simulink model "ScriptDemo"  (R2022b)
settings: configuration reference "TmVcThermal_Configuration_sub" (kept outside this file)
undefined symbols (not defined in the file or in its folder): aaaa, bbbb, cTmComprCtrl_D_u8HvacFlowTable_db, cTmComprCtrl_D_u8HvacFlowTable_sw, cTmComprCtrl_n_i16ChillCmpIMax, cTmComprCtrl_n_i16ChillCmpIMin, cTmComprCtrl_n_i16ChillCmpIMin666, cTmComprCtrl_n_i16ChillCmpPMax, cTmComprCtrl_n_i16ChillCmpPMin, cTmComprCtrl_n_i16CmpChillCoolRpmKiMax, cTmComprCtrl_n_i16CmpChillCoolRpmKiMin, cTmComprCtrl_n_i16CmpChillCoolRpmKpMax, cTmComprCtrl_n_i16CmpChillCoolRpmKpMin, cTmComprCtrl_n_i16CmpCoolRpmKiMax, cTmComprCtrl_n_i16CmpCoolRpmKiMin, cTmComprCtrl_n_i16CmpCoolRpmKpMax, cTmComprCtrl_n_i16CmpCoolRpmKpMin, cTmComprCtrl_n_i16SM4CmpHeatKiMax, cTmComprCtrl_n_i16SM4CmpHeatKiMin, cTmComprCtrl_n_i16SM4CmpHeatKpMax, cTmComprCtrl_n_i16SM4CmpHeatKpMin, cTmComprCtrl_n_i16SM5CmpHeatKiMax, cTmComprCtrl_n_i16SM5CmpHeatKiMin, cTmComprCtrl_n_i16SM5CmpHeatKpMax, cTmComprCtrl_n_i16SM5CmpHeatKpMin, cTmComprCtrl_n_i16SM6CmpHeatKiMax, cTmComprCtrl_n_i16SM6CmpHeatKiMin, cTmComprCtrl_n_i16SM6CmpHeatKpMax, cTmComprCtrl_n_i16SM6CmpHeatKpMin, cTmComprCtrl_n_u16CmpMaxSpdFanFltLimt, cTmComprCtrl_n_u16CmpMaxSpdLoSidePFltLimt, cTmComprCtrl_n_u16CmpMaxSpdSensorFltLimt, cTmComprCtrl_n_u16CompMinRpm, cTmComprCtrl_n_u16CompRpmIncThres, cTmComprCtrl_t_u16BattCooltFFPeriod, cTmComprCtrl_t_u16BattCooltPIPeriod, cTmComprCtrl_t_u16CmpCoolFFPeriod, cTmComprCtrl_t_u16CmpCoolPIPeriod, cTmComprCtrl_t_u16CoolCmpChillFFPeriod, cTmComprCtrl_t_u16CoolCmpChillPIPeriod, cTmComprCtrl_t_u16SM4CmpHeatFFPeriod, cTmComprCtrl_t_u16SM4CmpHeatPIPeriod, cTmComprCtrl_t_u16SM5CmpHeatFFPeriod, cTmComprCtrl_t_u16SM5CmpHeatPIPeriod, cTmComprCtrl_t_u16SM6CmpHeatFFPeriod, cTmComprCtrl_t_u16SM6CmpHeatPIPeriod, cTmComprCtrl_Te_EvapClearInteg, cTmComprCtrl_Te_i16HpReqTempSaturoffset, cTmComprCtrl_Te_i16SatLpReplaceDiff, cTmComprCtrl_Te_i16SM3BatDiffStartEvapDecOffset, cTmComprCtrl_Te_i16SM3EvapLo, cTmComprCtrl_Te_i16SM3TBatDiffEntEvapDecOffset, cTmComprCtrl_Te_i16SM3TBatDiffEntEvapDecOffsetQuit, cTmComprCtrl_Te_s32ErrCmpChillPIContinueCoolH, cTmComprCtrl_Te_s32ErrCmpChillPIContinueCoolL, cTmComprCtrl_Te_s32ErrCmpPIContinueChillH, cTmComprCtrl_Te_s32ErrCmpPIContinueChillL, cTmComprCtrl_Te_s32ErrCmpPIContinueCoolH, cTmComprCtrl_Te_s32ErrCmpPIContinueCoolL, cTmComprCtrl_Te_s32ErrCmpPIContinueHeatH ... (+398)
libraries: simulink x846, PCMULib x711, simulink_need_slupdate x4
(part 4 of 49)

== system ScriptDemo/Create/creatIFIn/After ==
  note: % 目的: 创建接口输入模型
      | % 限制: 本函数仅仅用于热系统autosar 系统， 运行函数前，需要提前加载生成arxml 对应的IDT文件
      | % 范例：creatIFIn('sheetNames',{'IF_InportsCommon','IF_InportsDiag','IF_Inports2F'})
  sVcCcm_Te_AmbTEstimd : Inport  OutputFunctionCall=on
  yVcCcm_B_AmbTEstimdQf : Inport  Port=2  OutDataTypeStr=boolean
  sVcCcm_Te_IncarTemp : Inport  Port=3
  sVcCcm_Qf_IncarTempQf : Inport  Port=4
  sVcCcm_Te_Evap : Inport  Port=5
  sVcCcm_Qf_TeEvap : Inport  Port=6
  yVcCcm_B_AirCondEnbl : Inport  Port=7  OutDataTypeStr=boolean
  sVcCcm_Te_EvapReq : Inport  Port=8
  yVcCcm_B_HvacHeatgReq : Inport  Port=9  OutDataTypeStr=boolean
  sVcCcm_Z_HvacAirMFlowEstimd : Inport  Port=10
  sVcCcm_Z_HexHeatrAirMFlowEstimd : Inport  Port=11
  sVcCcm_D_HvacFanSts : Inport  Port=12
  sVcCcm_X_ClimtRcirc : Inport  Port=13
  sVcCcm_X_HvacTFlpActlPosnFrtRowLe : Inport  Port=14
  sVcCcm_X_HvacTFlpActlPosnFrtRowRi : Inport  Port=15
  sVcCcm_Te_HeatrAirTReq : Inport  Port=16
  sVcCcm_Te_HvacHexAirT : Inport  Port=17
  yVcCcm_B_HvacHexAirTQf : Inport  Port=18  OutDataTypeStr=boolean
  yVcVdm_B_EcoClimaSts : Inport  Port=19  OutDataTypeStr=boolean
  Event_DTC_126A12_GetEventStatus : Inport  Port=20
  Event_DTC_126A14_GetEventStatus : Inport  Port=21
  Event_DTC_124314_GetEventStatus : Inport  Port=22
  Event_DTC_124312_GetEventStatus : Inport  Port=23
  Event_DTC_128D11_GetEventStatus : Inport  Port=24
  Event_DTC_128D15_GetEventStatus : Inport  Port=25
  Event_DTC_507011_GetEventStatus : Inport  Port=26
  Event_DTC_507015_GetEventStatus : Inport  Port=27
  Event_DTC_507111_GetEventStatus : Inport  Port=28
  Event_DTC_507115_GetEventStatus : Inport  Port=29
  Event_DTC_507C11_GetEventStatus : Inport  Port=30
  Event_DTC_507C15_GetEventStatus : Inport  Port=31
  Event_DTC_508C11_GetEventStatus : Inport  Port=32
  Event_DTC_508C15_GetEventStatus : Inport  Port=33
  Event_DTC_0A0011_GetEventStatus : Inport  Port=34
  Event_DTC_0A0015_GetEventStatus : Inport  Port=35
  Event_DTC_131F9C_GetEventStatus : Inport  Port=36
  Event_DTC_10687A_GetEventStatus : Inport  Port=37
  Event_DTC_91FF12_GetEventStatus : Inport  Port=38
  Event_DTC_91FF14_GetEventStatus : Inport  Port=39
  yGlAcHpM_B_HpmSov1Actv2FReq : Inport  Port=40  OutDataTypeStr=boolean
  yGlAcHpM_B_HpmSov1ActvCmd2F : Inport  Port=41  OutDataTypeStr=boolean
  yGlAcHpM_B_HpmSov2Actv2FReq : Inport  Port=42  OutDataTypeStr=boolean
  yGlAcHpM_B_HpmSov2ActvCmd2F : Inport  Port=43  OutDataTypeStr=boolean
  yGlAcHpM_B_HpmSov3Actv2FReq : Inport  Port=44  OutDataTypeStr=boolean
  yGlAcHpM_B_HpmSov3ActvCmd2F : Inport  Port=45  OutDataTypeStr=boolean
  yVcEac_B_ChillerValve2FReq : Inport  Port=46  OutDataTypeStr=boolean
  yVcEac_B_ChillerValveReq2F : Inport  Port=47  OutDataTypeStr=boolean
  yVcAc_B_EvaprVlvFrnt2FReq : Inport  Port=48  OutDataTypeStr=boolean
  yVcAc_B_EvaprVlvReqFrnt2F : Inport  Port=49  OutDataTypeStr=boolean
  yVcTmAf_B_FanPwm2FReq : Inport  Port=50  OutDataTypeStr=boolean
  sVcTmAf_X_FanPwmReq2F : Inport  Port=51
  yGlTmHgMgt_B_PTCPumpSpd2FReq : Inport  Port=52  OutDataTypeStr=boolean
  sGlTmHgMgt_X_PTCPumpSpdReq2F : Inport  Port=53
  yGlHwDrvDiag_B_BattPmp2FReq : Inport  Port=54  OutDataTypeStr=boolean
  sGlTmBcc_X_BattCooltPmpReq2F : Inport  Port=55
  yVcTmHcc_B_EmCooltPmp2FReq : Inport  Port=56  OutDataTypeStr=boolean
  sVcTmHcc_X_EmCooltPmpReq2F : Inport  Port=57
  yVcBctv_B_VlvPos2FReq : Inport  Port=58  OutDataTypeStr=boolean
  sVcBctv_X_VlvPosReq2F : Inport  Port=59
  TmIn : Subsystem
  wires:
  TmIn/1(sTmIn_Te_s32AmbTEstimd) -> [sTmIn_Te_s32AmbTEstimd]
  TmIn/2(yTmIn_B_AmbTEstimdQf) -> [yTmIn_B_AmbTEstimdQf]
  TmIn/3(sTmIn_Te_s32IncarTemp) -> [sTmIn_Te_s32IncarTemp]
  TmIn/4(sTmIn_D_u8IncarTempQf) -> [sTmIn_D_u8IncarTempQf]
  TmIn/5(sTmIn_Te_s32Evap) -> [sTmIn_Te_s32Evap]
  TmIn/6(yTmIn_B_TeEvap) -> [yTmIn_B_TeEvap]
  TmIn/7(yTmIn_B_AirCondEnbl) -> [yTmIn_B_AirCondEnbl]
  TmIn/8(sTmIn_Te_s32EvapReq) -> [sTmIn_Te_s32EvapReq]
  TmIn/9(yTmIn_B_HvacHeatgReq) -> [yTmIn_B_HvacHeatgReq]
  TmIn/10(sTmIn_md_s32HvacAirMFlowEstimd) -> [sTmIn_md_s32HvacAirMFlowEstimd]
  TmIn/11(sTmIn_md_s32HexHeatrAirMFlowEstimd) -> [sTmIn_md_s32HexHeatrAirMFlowEstimd]
  TmIn/12(sTmIn_D_u8HvacFanSts) -> [sTmIn_D_u8HvacFanSts]
  TmIn/13(sTmIn_X_s32ClimtRcirc) -> [sTmIn_X_s32ClimtRcirc]
  TmIn/14(sTmIn_X_s32HvacTFlpActlPosnFrtRowLe) -> [sTmIn_X_s32HvacTFlpActlPosnFrtRowLe]
  TmIn/15(sTmIn_X_s32HvacTFlpActlPosnFrtRowRi) -> [sTmIn_X_s32HvacTFlpActlPosnFrtRowRi]
  TmIn/16(sTmIn_Te_s32HeatrAirTReq) -> [sTmIn_Te_s32HeatrAirTReq]
  TmIn/17(sTmIn_Te_s32HvacHexAirT) -> [sTmIn_Te_s32HvacHexAirT]
  TmIn/18(yTmIn_B_HvacHexAirTQf) -> [yTmIn_B_HvacHexAirTQf]
  TmIn/19(yTmIn_B_EcoClimaSts) -> [yTmIn_B_EcoClimaSts]
  TmIn/20(sTmIn_D_u8VcEvLoSidePSB) -> [sTmIn_D_u8VcEvLoSidePSB]
  TmIn/21(sTmIn_D_u8VcEvLoSidePOP) -> [sTmIn_D_u8VcEvLoSidePOP]
  TmIn/22(sTmIn_D_u8VcEvHiSidePOP) -> [sTmIn_D_u8VcEvHiSidePOP]
  TmIn/23(sTmIn_D_u8VcEvHiSidePSB) -> [sTmIn_D_u8VcEvHiSidePSB]
  TmIn/24(sTmIn_D_u8VcEvHiSideTmpSnrSG) -> [sTmIn_D_u8VcEvHiSideTmpSnrSG]
  TmIn/25(sTmIn_D_u8VcEvOutrCondOutTOP) -> [sTmIn_D_u8VcEvOutrCondOutTOP]
  TmIn/26(sTmIn_D_u8VcEvChillerOutTSG) -> [sTmIn_D_u8VcEvChillerOutTSG]
  TmIn/27(sTmIn_D_u8VcEvChillerOutTOP) -> [sTmIn_D_u8VcEvChillerOutTOP]
  TmIn/28(sTmIn_D_u8VcEvInrCondOutTSG) -> [sTmIn_D_u8VcEvInrCondOutTSG]
  TmIn/29(sTmIn_D_u8VcEvInrCondOutTOP) -> [sTmIn_D_u8VcEvInrCondOutTOP]
  TmIn/30(sTmIn_D_u8VcEvEvapOutTSG) -> [sTmIn_D_u8VcEvEvapOutTSG]
  TmIn/31(sTmIn_D_u8VcEvEvapOutTOP) -> [sTmIn_D_u8VcEvEvapOutTOP]
  TmIn/32(sTmIn_D_u8VcEvCmprDischrgTSG) -> [sTmIn_D_u8VcEvCmprDischrgTSG]
  TmIn/33(sTmIn_D_u8VcEvCmprDischrgTOP) -> [sTmIn_D_u8VcEvCmprDischrgTOP]
  TmIn/34(sTmIn_D_u8VcEvTmpClSrSG) -> [sTmIn_D_u8VcEvTmpClSrSG]
  TmIn/35(sTmIn_D_u8VcEvTmpClSrOP) -> [sTmIn_D_u8VcEvTmpClSrOP]
  TmIn/36(sTmIn_D_u8VcEvELDTCooltLvlLo) -> [sTmIn_D_u8VcEvELDTCooltLvlLo]
  TmIn/37(sTmIn_D_u8VcEvBattCooltLvlLo) -> [sTmIn_D_u8VcEvBattCooltLvlLo]
  TmIn/38(sTmIn_D_u8VcEvNoHpHighSidePSnrSB) -> [sTmIn_D_u8VcEvNoHpHighSidePSnrSB]
  TmIn/39(sTmIn_D_u8VcEvNoHpHighSidePSnrOP) -> [sTmIn_D_u8VcEvNoHpHighSidePSnrOP]
  TmIn/40(yTmIn_B_HpmSov1Actv2FReq) -> [yTmIn_B_HpmSov1Actv2FReq]
  TmIn/41(yTmIn_B_HpmSov1ActvCmd2F) -> [yTmIn_B_HpmSov1ActvCmd2F]
  TmIn/42(yTmIn_B_HpmSov2Actv2FReq) -> [yTmIn_B_HpmSov2Actv2FReq]
  TmIn/43(yTmIn_B_HpmSov2ActvCmd2F) -> [yTmIn_B_HpmSov2ActvCmd2F]
  TmIn/44(yTmIn_B_HpmSov3Actv2FReq) -> [yTmIn_B_HpmSov3Actv2FReq]
  TmIn/45(yTmIn_B_HpmSov3ActvCmd2F) -> [yTmIn_B_HpmSov3ActvCmd2F]
  TmIn/46(yTmIn_B_ChillerValve2FReq) -> [yTmIn_B_ChillerValve2FReq]
  TmIn/47(yTmIn_B_ChillerValveReq2F) -> [yTmIn_B_ChillerValveReq2F]
  TmIn/48(yTmIn_B_EvaprVlvFrnt2FReq) -> [yTmIn_B_EvaprVlvFrnt2FReq]
  TmIn/49(yTmIn_B_EvaprVlvReqFrnt2F) -> [yTmIn_B_EvaprVlvReqFrnt2F]
  TmIn/50(yTmIn_B_FanPwm2FReq) -> [yTmIn_B_FanPwm2FReq]
  TmIn/51(sTmIn_X_s32FanPwmReq2F) -> [sTmIn_X_s32FanPwmReq2F]
  TmIn/52(yTmIn_B_PTCPumpSpd2FReq) -> [yTmIn_B_PTCPumpSpd2FReq]
  TmIn/53(sTmIn_X_s32PTCPumpSpdReq2F) -> [sTmIn_X_s32PTCPumpSpdReq2F]
  TmIn/54(yTmIn_B_BattPmp2FReq) -> [yTmIn_B_BattPmp2FReq]
  TmIn/55(sTmIn_X_s32BattCooltPmpReq2F) -> [sTmIn_X_s32BattCooltPmpReq2F]
  TmIn/56(yTmIn_B_EmCooltPmp2FReq) -> [yTmIn_B_EmCooltPmp2FReq]
  TmIn/57(sTmIn_X_s32EmCooltPmpReq2F) -> [sTmIn_X_s32EmCooltPmpReq2F]
  TmIn/58(yTmIn_B_BctvVlvPos2FReq) -> [yTmIn_B_BctvVlvPos2FReq]
  TmIn/59(sTmIn_X_u8BctvVlvPosReq2F) -> [sTmIn_X_u8BctvVlvPosReq2F]
  sVcCcm_Te_AmbTEstimd/1 -> TmIn/1(sVcCcm_Te_AmbTEstimd)
  yVcCcm_B_AmbTEstimdQf/1 -> TmIn/2(yVcCcm_B_AmbTEstimdQf)
  sVcCcm_Te_IncarTemp/1 -> TmIn/3(sVcCcm_Te_IncarTemp)
  sVcCcm_Qf_IncarTempQf/1 -> TmIn/4(sVcCcm_Qf_IncarTempQf)
  sVcCcm_Te_Evap/1 -> TmIn/5(sVcCcm_Te_Evap)
  sVcCcm_Qf_TeEvap/1 -> TmIn/6(sVcCcm_Qf_TeEvap)
  yVcCcm_B_AirCondEnbl/1 -> TmIn/7(yVcCcm_B_AirCondEnbl)
  sVcCcm_Te_EvapReq/1 -> TmIn/8(sVcCcm_Te_EvapReq)
  yVcCcm_B_HvacHeatgReq/1 -> TmIn/9(yVcCcm_B_HvacHeatgReq)
  sVcCcm_Z_HvacAirMFlowEstimd/1 -> TmIn/10(sVcCcm_Z_HvacAirMFlowEstimd)
  sVcCcm_Z_HexHeatrAirMFlowEstimd/1 -> TmIn/11(sVcCcm_Z_HexHeatrAirMFlowEstimd)
  sVcCcm_D_HvacFanSts/1 -> TmIn/12(sVcCcm_D_HvacFanSts)
  sVcCcm_X_ClimtRcirc/1 -> TmIn/13(sVcCcm_X_ClimtRcirc)
  sVcCcm_X_HvacTFlpActlPosnFrtRowLe/1 -> TmIn/14(sVcCcm_X_HvacTFlpActlPosnFrtRowLe)
  sVcCcm_X_HvacTFlpActlPosnFrtRowRi/1 -> TmIn/15(sVcCcm_X_HvacTFlpActlPosnFrtRowRi)
  sVcCcm_Te_HeatrAirTReq/1 -> TmIn/16(sVcCcm_Te_HeatrAirTReq)
  sVcCcm_Te_HvacHexAirT/1 -> TmIn/17(sVcCcm_Te_HvacHexAirT)
  yVcCcm_B_HvacHexAirTQf/1 -> TmIn/18(yVcCcm_B_HvacHexAirTQf)
  yVcVdm_B_EcoClimaSts/1 -> TmIn/19(yVcVdm_B_EcoClimaSts)
  Event_DTC_126A12_GetEventStatus/1 -> TmIn/20(Event_DTC_126A12_GetEventStatus)
  Event_DTC_126A14_GetEventStatus/1 -> TmIn/21(Event_DTC_126A14_GetEventStatus)
  Event_DTC_124314_GetEventStatus/1 -> TmIn/22(Event_DTC_124314_GetEventStatus)
  Event_DTC_124312_GetEventStatus/1 -> TmIn/23(Event_DTC_124312_GetEventStatus)
  Event_DTC_128D11_GetEventStatus/1 -> TmIn/24(Event_DTC_128D11_GetEventStatus)
  Event_DTC_128D15_GetEventStatus/1 -> TmIn/25(Event_DTC_128D15_GetEventStatus)
  Event_DTC_507011_GetEventStatus/1 -> TmIn/26(Event_DTC_507011_GetEventStatus)
  Event_DTC_507015_GetEventStatus/1 -> TmIn/27(Event_DTC_507015_GetEventStatus)
  Event_DTC_507111_GetEventStatus/1 -> TmIn/28(Event_DTC_507111_GetEventStatus)
  Event_DTC_507115_GetEventStatus/1 -> TmIn/29(Event_DTC_507115_GetEventStatus)
  Event_DTC_507C11_GetEventStatus/1 -> TmIn/30(Event_DTC_507C11_GetEventStatus)
  Event_DTC_507C15_GetEventStatus/1 -> TmIn/31(Event_DTC_507C15_GetEventStatus)
  Event_DTC_508C11_GetEventStatus/1 -> TmIn/32(Event_DTC_508C11_GetEventStatus)
  Event_DTC_508C15_GetEventStatus/1 -> TmIn/33(Event_DTC_508C15_GetEventStatus)
  Event_DTC_0A0011_GetEventStatus/1 -> TmIn/34(Event_DTC_0A0011_GetEventStatus)
  Event_DTC_0A0015_GetEventStatus/1 -> TmIn/35(Event_DTC_0A0015_GetEventStatus)
  Event_DTC_131F9C_GetEventStatus/1 -> TmIn/36(Event_DTC_131F9C_GetEventStatus)
  Event_DTC_10687A_GetEventStatus/1 -> TmIn/37(Event_DTC_10687A_GetEventStatus)
  Event_DTC_91FF12_GetEventStatus/1 -> TmIn/38(Event_DTC_91FF12_GetEventStatus)
  Event_DTC_91FF14_GetEventStatus/1 -> TmIn/39(Event_DTC_91FF14_GetEventStatus)
  yGlAcHpM_B_HpmSov1Actv2FReq/1 -> TmIn/40(yGlAcHpM_B_HpmSov1Actv2FReq)
  yGlAcHpM_B_HpmSov1ActvCmd2F/1 -> TmIn/41(yGlAcHpM_B_HpmSov1ActvCmd2F)
  yGlAcHpM_B_HpmSov2Actv2FReq/1 -> TmIn/42(yGlAcHpM_B_HpmSov2Actv2FReq)
  yGlAcHpM_B_HpmSov2ActvCmd2F/1 -> TmIn/43(yGlAcHpM_B_HpmSov2ActvCmd2F)
  yGlAcHpM_B_HpmSov3Actv2FReq/1 -> TmIn/44(yGlAcHpM_B_HpmSov3Actv2FReq)
  yGlAcHpM_B_HpmSov3ActvCmd2F/1 -> TmIn/45(yGlAcHpM_B_HpmSov3ActvCmd2F)
  yVcEac_B_ChillerValve2FReq/1 -> TmIn/46(yVcEac_B_ChillerValve2FReq)
  yVcEac_B_ChillerValveReq2F/1 -> TmIn/47(yVcEac_B_ChillerValveReq2F)
  yVcAc_B_EvaprVlvFrnt2FReq/1 -> TmIn/48(yVcAc_B_EvaprVlvFrnt2FReq)
  yVcAc_B_EvaprVlvReqFrnt2F/1 -> TmIn/49(yVcAc_B_EvaprVlvReqFrnt2F)
  yVcTmAf_B_FanPwm2FReq/1 -> TmIn/50(yVcTmAf_B_FanPwm2FReq)
  sVcTmAf_X_FanPwmReq2F/1 -> TmIn/51(sVcTmAf_X_FanPwmReq2F)
  yGlTmHgMgt_B_PTCPumpSpd2FReq/1 -> TmIn/52(yGlTmHgMgt_B_PTCPumpSpd2FReq)
  sGlTmHgMgt_X_PTCPumpSpdReq2F/1 -> TmIn/53(sGlTmHgMgt_X_PTCPumpSpdReq2F)
  yGlHwDrvDiag_B_BattPmp2FReq/1 -> TmIn/54(yGlHwDrvDiag_B_BattPmp2FReq)
  sGlTmBcc_X_BattCooltPmpReq2F/1 -> TmIn/55(sGlTmBcc_X_BattCooltPmpReq2F)
  yVcTmHcc_B_EmCooltPmp2FReq/1 -> TmIn/56(yVcTmHcc_B_EmCooltPmp2FReq)
  sVcTmHcc_X_EmCooltPmpReq2F/1 -> TmIn/57(sVcTmHcc_X_EmCooltPmpReq2F)
  yVcBctv_B_VlvPos2FReq/1 -> TmIn/58(yVcBctv_B_VlvPos2FReq)
  sVcBctv_X_VlvPosReq2F/1 -> TmIn/59(sVcBctv_X_VlvPosReq2F)

== system ScriptDemo/Create/creatIFIn/Before ==

== system ScriptDemo/Create/creatIFOut/After ==
  note: % 目的: 创建接口输出模型
      | % 限制: 本函数仅仅用于热系统autosar 系统， 运行函数前，需要提前加载生成arxml 对应的IDT文件
      | % 范例：creatIFOut('sheetNames',{'IF_OutportsCommon','IF_OutportsDiag','IF_Outports2F'})
  TmOut : Subsystem
  sVcEac_n_ElacCmprReq : Outport
  sVcEac_D_ElacCmprRelease : Outport  Port=2
  sVcEac_Pw_ElacCmprMax : Outport  Port=3
  sGlTmEexv_X_VlvPosReq : Outport  Port=4
  yGlTmEexv_B_PosnHeatdReq : Outport  Port=5  OutDataTypeStr=boolean
  yGlTmEexv_B_PosnCalibReq : Outport  Port=6  OutDataTypeStr=boolean
  yGlTmEexv_B_PosnMovEnable : Outport  Port=7  OutDataTypeStr=boolean
  sGlTmBexv_X_VlvPosReq : Outport  Port=8
  yGlTmBexv_B_PosnCalibReq : Outport  Port=9  OutDataTypeStr=boolean
  yGlTmBexv_B_PosnHeatdReq : Outport  Port=10  OutDataTypeStr=boolean
  yGlTmBexv_B_PosnMovEnable : Outport  Port=11  OutDataTypeStr=boolean
  sGlTmCexv_X_VlvPosReq : Outport  Port=12
  yGlTmCexv_B_PosnCalibReq : Outport  Port=13  OutDataTypeStr=boolean
  yGlTmCexv_B_PosnHeatdReq : Outport  Port=14  OutDataTypeStr=boolean
  yGlTmCexv_B_PosnMovEnable : Outport  Port=15  OutDataTypeStr=boolean
  sGlTmBctv_D_VlvRefDrvReq : Outport  Port=16
  sGlTmBctv_D_VlvActvSaveReq : Outport  Port=17
  sGlTmBctv_X_VlvPosReq : Outport  Port=18
  sGlTmBctv_D_VlvSpdLvlReq : Outport  Port=19
  sGlTmBcfv_D_VlvRefDrvReq : Outport  Port=20
  sGlTmDiag_D_EventDTC126A12 : Outport  Port=21
  sGlTmDiag_D_EventDTC126A14 : Outport  Port=22
  sGlTmDiag_D_EventDTC124314 : Outport  Port=23
  sGlTmDiag_D_EventDTC124312 : Outport  Port=24
  sGlTmDiag_D_EventDTC128D11 : Outport  Port=25
  sGlTmDiag_D_EventDTC128D15 : Outport  Port=26
  sGlTmDiag_D_EventDTC10687A : Outport  Port=27
  sGlTmDiag_D_EventDTC976612 : Outport  Port=28
  sGlTmDiag_D_EventDTC976712 : Outport  Port=29
  sGlTmDiag_D_EventDTC979012 : Outport  Port=30
  sGlTmDiag_D_EventDTC129B12 : Outport  Port=31
  sGlTmDiag_D_EventDTC979112 : Outport  Port=32
  sGlTmDiag_D_EventDTC92FE12 : Outport  Port=33
  sGlTmDiag_D_EventDTC92FE13 : Outport  Port=34
  sGlTmDiag_D_EventDTC92FE11 : Outport  Port=35
  sGlTmDiag_D_EventDTC92FEA1 : Outport  Port=36
  sGlTmDiag_D_EventDTC92FE71 : Outport  Port=37
  sGlTmDiag_D_EventDTC92FE04 : Outport  Port=38
  sGlTmDiag_D_EventDTC92A612 : Outport  Port=39
  sGlTmDiag_D_EventDTC92A613 : Outport  Port=40
  sGlAcHpM_D_HpmSov1Actv2FEnState : Outport  Port=41
  sGlAcHpM_D_HpmSov2Actv2FEnState : Outport  Port=42
  sGlAcHpM_D_HpmSov3Actv2FEnState : Outport  Port=43
  sVcTmAf_D_FanPwm2FEnState : Outport  Port=44
  sGlTmBcc_D_BattCooltPmp2FEnState : Outport  Port=45
  sVcTmHcc_D_EmCooltPmp2FEnState : Outport  Port=46
  sGlTmHgMgt_D_PTCPumpSpd2FEnState : Outport  Port=47
  sVcEctv_D_VlvMoveEna2FEnaState : Outport  Port=48
  sVcEctv_D_VlvPos2FEnaState : Outport  Port=49
  sVcBctv_D_VlvRef2FEnaState : Outport  Port=50
  sVcBctv_D_VlvPos2FEnaState : Outport  Port=51
  sVcBcfv_D_VlvRef2FEnaState : Outport  Port=52
  sVcBcfv_D_VlvPos2FEnaState : Outport  Port=53
  sVcBexv_D_ExvCal2FEnaState : Outport  Port=54
  sVcBexv_D_ExvMoveEna2FEnaState : Outport  Port=55
  sVcBexv_D_ExvPosnReq2FEnaState : Outport  Port=56
  sVcCexv_D_ExvCal2FEnaState : Outport  Port=57
  sVcCexv_D_ExvMoveEna2FEnaState : Outport  Port=58
  sVcCexv_D_ExvPosnReq2FEnaState : Outport  Port=59
  sVcEexv_D_ExvCal2FEnaState : Outport  Port=60
  wires:
  [sTmOut_n_u16ElacCmprReq] -> TmOut/1(sTmOut_n_u16ElacCmprReq)
  [sTmOut_D_u8ElacCmprRelease] -> TmOut/2(sTmOut_D_u8ElacCmprRelease)
  [sTmOut_Pw_s32ElacCmprMax] -> TmOut/3(sTmOut_Pw_s32ElacCmprMax)
  [sTmOut_X_s32EexvVlvPosReq] -> TmOut/4(sTmOut_X_s32EexvVlvPosReq)
  [yTmOut_B_EexvPosnCalibReq] -> TmOut/5(yTmOut_B_EexvPosnCalibReq)
  [yTmOut_B_EexvPosnMovEnable] -> TmOut/6(yTmOut_B_EexvPosnMovEnable)
  [sTmOut_X_s32BexvVlvPosReq] -> TmOut/7(sTmOut_X_s32BexvVlvPosReq)
  [yTmOut_B_BexvPosnCalibReq] -> TmOut/8(yTmOut_B_BexvPosnCalibReq)
  [yTmOut_B_BexvPosnMovEnable] -> TmOut/9(yTmOut_B_BexvPosnMovEnable)
  [sTmOut_X_s32CexvVlvPosReq] -> TmOut/10(sTmOut_X_s32CexvVlvPosReq)
  [yTmOut_B_CexvPosnCalibReq] -> TmOut/11(yTmOut_B_CexvPosnCalibReq)
  [yTmOut_B_CexvPosnMovEnable] -> TmOut/12(yTmOut_B_CexvPosnMovEnable)
  [sTmOut_D_u8BctvVlvRefDrvReq] -> TmOut/13(sTmOut_D_u8BctvVlvRefDrvReq)
  [sTmOut_X_u8BctvVlvPosReq] -> TmOut/14(sTmOut_X_u8BctvVlvPosReq)
  [sTmOut_D_u8BcfvVlvRefDrvReq] -> TmOut/15(sTmOut_D_u8BcfvVlvRefDrvReq)
  [sTmOut_D_u8VcEvLowSidePSnrSB] -> TmOut/16(sTmOut_D_u8VcEvLowSidePSnrSB)
  [sTmOut_D_u8VcEvLowSidePSnrOP] -> TmOut/17(sTmOut_D_u8VcEvLowSidePSnrOP)
  [sTmOut_D_u8VcEvHiSidePSnrOP] -> TmOut/18(sTmOut_D_u8VcEvHiSidePSnrOP)
  [sTmOut_D_u8VcEvHiSidePSnrSB] -> TmOut/19(sTmOut_D_u8VcEvHiSidePSnrSB)
  [sTmOut_D_u8VcEvHiSideTmpSnrSG] -> TmOut/20(sTmOut_D_u8VcEvHiSideTmpSnrSG)
  [sTmOut_D_u8VcEvHiSideTmpSnrOP] -> TmOut/21(sTmOut_D_u8VcEvHiSideTmpSnrOP)
  [sTmOut_D_u8VcEvBattCooltLvlLo] -> TmOut/22(sTmOut_D_u8VcEvBattCooltLvlLo)
  [sTmOut_D_u8VcEvSov1SB] -> TmOut/23(sTmOut_D_u8VcEvSov1SB)
  [sTmOut_D_u8VcEvSov2SB] -> TmOut/24(sTmOut_D_u8VcEvSov2SB)
  [sTmOut_D_u8VcEvSov3SB] -> TmOut/25(sTmOut_D_u8VcEvSov3SB)
  [sTmOut_D_u8VcEvSov5SB] -> TmOut/26(sTmOut_D_u8VcEvSov5SB)
  [sTmOut_D_u8VcEvSov4SB] -> TmOut/27(sTmOut_D_u8VcEvSov4SB)
  [sTmOut_D_u8VcEvSBFan] -> TmOut/28(sTmOut_D_u8VcEvSBFan)
  [sTmOut_D_u8VcEvOPFan] -> TmOut/29(sTmOut_D_u8VcEvOPFan)
  [sTmOut_D_u8VcEvSGFan] -> TmOut/30(sTmOut_D_u8VcEvSGFan)
  [sTmOut_D_u8VcEvVolErrFan] -> TmOut/31(sTmOut_D_u8VcEvVolErrFan)
  [sTmOut_D_u8VcEvBlokFan] -> TmOut/32(sTmOut_D_u8VcEvBlokFan)
  [sTmOut_D_u8VcEvCircutInteFlt] -> TmOut/33(sTmOut_D_u8VcEvCircutInteFlt)
  [sTmOut_D_u8VcEvHmPumpSB] -> TmOut/34(sTmOut_D_u8VcEvHmPumpSB)
  [sTmOut_D_u8VcEvHmPumpOC] -> TmOut/35(sTmOut_D_u8VcEvHmPumpOC)
  [sTmOut_D_u8HpmSov1Actv2FEnState] -> TmOut/36(sTmOut_D_u8HpmSov1Actv2FEnState)
  [sTmOut_D_u8HpmSov2Actv2FEnState] -> TmOut/37(sTmOut_D_u8HpmSov2Actv2FEnState)
  [sTmOut_D_u8HpmSov3Actv2FEnState] -> TmOut/38(sTmOut_D_u8HpmSov3Actv2FEnState)
  [sTmOut_D_u8FanPwm2FEnState] -> TmOut/39(sTmOut_D_u8FanPwm2FEnState)
  [sTmOut_D_u8BattCooltPmp2FEnState] -> TmOut/40(sTmOut_D_u8BattCooltPmp2FEnState)
  [sTmOut_D_u8EmCooltPmp2FEnState] -> TmOut/41(sTmOut_D_u8EmCooltPmp2FEnState)
  [sTmOut_D_u8PTCPumpSpd2FEnState] -> TmOut/42(sTmOut_D_u8PTCPumpSpd2FEnState)
  [sTmOut_D_u8EctvVlvMoveEna2FEnaState] -> TmOut/43(sTmOut_D_u8EctvVlvMoveEna2FEnaState)
  [sTmOut_D_u8EctvVlvPos2FEnaState] -> TmOut/44(sTmOut_D_u8EctvVlvPos2FEnaState)
  [sTmOut_D_u8BctvVlvRef2FEnaState] -> TmOut/45(sTmOut_D_u8BctvVlvRef2FEnaState)
  [sTmOut_D_u8BctvVlvPos2FEnaState] -> TmOut/46(sTmOut_D_u8BctvVlvPos2FEnaState)
  [sTmOut_D_u8BcfvVlvRef2FEnaState] -> TmOut/47(sTmOut_D_u8BcfvVlvRef2FEnaState)
  [sTmOut_D_u8BcfvVlvPos2FEnaState] -> TmOut/48(sTmOut_D_u8BcfvVlvPos2FEnaState)
  [sTmOut_D_u8BexvCal2FEnaState] -> TmOut/49(sTmOut_D_u8BexvCal2FEnaState)
  [sTmOut_D_u8BexvMoveEna2FEnaState] -> TmOut/50(sTmOut_D_u8BexvMoveEna2FEnaState)
  [sTmOut_D_u8BexvPosnReq2FEnaState] -> TmOut/51(sTmOut_D_u8BexvPosnReq2FEnaState)
  [sTmOut_D_u8CexvCal2FEnaState] -> TmOut/52(sTmOut_D_u8CexvCal2FEnaState)
  [sTmOut_D_u8CexvMoveEna2FEnaState] -> TmOut/53(sTmOut_D_u8CexvMoveEna2FEnaState)
  [sTmOut_D_u8CexvPosnReq2FEnaState] -> TmOut/54(sTmOut_D_u8CexvPosnReq2FEnaState)
  [sTmOut_D_u8EexvCal2FEnaState] -> TmOut/55(sTmOut_D_u8EexvCal2FEnaState)
  TmOut/1(sVcEac_n_ElacCmprReq) -> sVcEac_n_ElacCmprReq/1
  TmOut/2(sVcEac_D_ElacCmprRelease) -> sVcEac_D_ElacCmprRelease/1
  TmOut/3(sVcEac_Pw_ElacCmprMax) -> sVcEac_Pw_ElacCmprMax/1
  TmOut/4(sGlTmEexv_X_VlvPosReq) -> sGlTmEexv_X_VlvPosReq/1
  TmOut/5(yGlTmEexv_B_PosnHeatdReq) -> yGlTmEexv_B_PosnHeatdReq/1
  TmOut/6(yGlTmEexv_B_PosnCalibReq) -> yGlTmEexv_B_PosnCalibReq/1
  TmOut/7(yGlTmEexv_B_PosnMovEnable) -> yGlTmEexv_B_PosnMovEnable/1
  TmOut/8(sGlTmBexv_X_VlvPosReq) -> sGlTmBexv_X_VlvPosReq/1
  TmOut/9(yGlTmBexv_B_PosnCalibReq) -> yGlTmBexv_B_PosnCalibReq/1
  TmOut/10(yGlTmBexv_B_PosnHeatdReq) -> yGlTmBexv_B_PosnHeatdReq/1
  TmOut/11(yGlTmBexv_B_PosnMovEnable) -> yGlTmBexv_B_PosnMovEnable/1
  TmOut/12(sGlTmCexv_X_VlvPosReq) -> sGlTmCexv_X_VlvPosReq/1
  TmOut/13(yGlTmCexv_B_PosnCalibReq) -> yGlTmCexv_B_PosnCalibReq/1
  TmOut/14(yGlTmCexv_B_PosnHeatdReq) -> yGlTmCexv_B_PosnHeatdReq/1
  TmOut/15(yGlTmCexv_B_PosnMovEnable) -> yGlTmCexv_B_PosnMovEnable/1
  TmOut/16(sGlTmBctv_D_VlvRefDrvReq) -> sGlTmBctv_D_VlvRefDrvReq/1
  TmOut/17(sGlTmBctv_D_VlvActvSaveReq) -> sGlTmBctv_D_VlvActvSaveReq/1
  TmOut/18(sGlTmBctv_X_VlvPosReq) -> sGlTmBctv_X_VlvPosReq/1
  TmOut/19(sGlTmBctv_D_VlvSpdLvlReq) -> sGlTmBctv_D_VlvSpdLvlReq/1
  TmOut/20(sGlTmBcfv_D_VlvRefDrvReq) -> sGlTmBcfv_D_VlvRefDrvReq/1
  TmOut/21(sGlTmDiag_D_EventDTC126A12) -> sGlTmDiag_D_EventDTC126A12/1
  TmOut/22(sGlTmDiag_D_EventDTC126A14) -> sGlTmDiag_D_EventDTC126A14/1
  TmOut/23(sGlTmDiag_D_EventDTC124314) -> sGlTmDiag_D_EventDTC124314/1
  TmOut/24(sGlTmDiag_D_EventDTC124312) -> sGlTmDiag_D_EventDTC124312/1
  TmOut/25(sGlTmDiag_D_EventDTC128D11) -> sGlTmDiag_D_EventDTC128D11/1
  TmOut/26(sGlTmDiag_D_EventDTC128D15) -> sGlTmDiag_D_EventDTC128D15/1
  TmOut/27(sGlTmDiag_D_EventDTC10687A) -> sGlTmDiag_D_EventDTC10687A/1
  TmOut/28(sGlTmDiag_D_EventDTC976612) -> sGlTmDiag_D_EventDTC976612/1
  TmOut/29(sGlTmDiag_D_EventDTC976712) -> sGlTmDiag_D_EventDTC976712/1
  TmOut/30(sGlTmDiag_D_EventDTC979012) -> sGlTmDiag_D_EventDTC979012/1
  TmOut/31(sGlTmDiag_D_EventDTC129B12) -> sGlTmDiag_D_EventDTC129B12/1
  TmOut/32(sGlTmDiag_D_EventDTC979112) -> sGlTmDiag_D_EventDTC979112/1
  TmOut/33(sGlTmDiag_D_EventDTC92FE12) -> sGlTmDiag_D_EventDTC92FE12/1
  TmOut/34(sGlTmDiag_D_EventDTC92FE13) -> sGlTmDiag_D_EventDTC92FE13/1
  TmOut/35(sGlTmDiag_D_EventDTC92FE11) -> sGlTmDiag_D_EventDTC92FE11/1
  TmOut/36(sGlTmDiag_D_EventDTC92FEA1) -> sGlTmDiag_D_EventDTC92FEA1/1
  TmOut/37(sGlTmDiag_D_EventDTC92FE71) -> sGlTmDiag_D_EventDTC92FE71/1
  TmOut/38(sGlTmDiag_D_EventDTC92FE04) -> sGlTmDiag_D_EventDTC92FE04/1
  TmOut/39(sGlTmDiag_D_EventDTC92A612) -> sGlTmDiag_D_EventDTC92A612/1
  TmOut/40(sGlTmDiag_D_EventDTC92A613) -> sGlTmDiag_D_EventDTC92A613/1
  TmOut/41(sGlAcHpM_D_HpmSov1Actv2FEnState) -> sGlAcHpM_D_HpmSov1Actv2FEnState/1
  TmOut/42(sGlAcHpM_D_HpmSov2Actv2FEnState) -> sGlAcHpM_D_HpmSov2Actv2FEnState/1
  TmOut/43(sGlAcHpM_D_HpmSov3Actv2FEnState) -> sGlAcHpM_D_HpmSov3Actv2FEnState/1
  TmOut/44(sVcTmAf_D_FanPwm2FEnState) -> sVcTmAf_D_FanPwm2FEnState/1
  TmOut/45(sGlTmBcc_D_BattCooltPmp2FEnState) -> sGlTmBcc_D_BattCooltPmp2FEnState/1
  TmOut/46(sVcTmHcc_D_EmCooltPmp2FEnState) -> sVcTmHcc_D_EmCooltPmp2FEnState/1
  TmOut/47(sGlTmHgMgt_D_PTCPumpSpd2FEnState) -> sGlTmHgMgt_D_PTCPumpSpd2FEnState/1
  TmOut/48(sVcEctv_D_VlvMoveEna2FEnaState) -> sVcEctv_D_VlvMoveEna2FEnaState/1
  TmOut/49(sVcEctv_D_VlvPos2FEnaState) -> sVcEctv_D_VlvPos2FEnaState/1
  TmOut/50(sVcBctv_D_VlvRef2FEnaState) -> sVcBctv_D_VlvRef2FEnaState/1
  TmOut/51(sVcBctv_D_VlvPos2FEnaState) -> sVcBctv_D_VlvPos2FEnaState/1
  TmOut/52(sVcBcfv_D_VlvRef2FEnaState) -> sVcBcfv_D_VlvRef2FEnaState/1
  TmOut/53(sVcBcfv_D_VlvPos2FEnaState) -> sVcBcfv_D_VlvPos2FEnaState/1
  TmOut/54(sVcBexv_D_ExvCal2FEnaState) -> sVcBexv_D_ExvCal2FEnaState/1
  TmOut/55(sVcBexv_D_ExvMoveEna2FEnaState) -> sVcBexv_D_ExvMoveEna2FEnaState/1
  TmOut/56(sVcBexv_D_ExvPosnReq2FEnaState) -> sVcBexv_D_ExvPosnReq2FEnaState/1
  TmOut/57(sVcCexv_D_ExvCal2FEnaState) -> sVcCexv_D_ExvCal2FEnaState/1
  TmOut/58(sVcCexv_D_ExvMoveEna2FEnaState) -> sVcCexv_D_ExvMoveEna2FEnaState/1
  TmOut/59(sVcCexv_D_ExvPosnReq2FEnaState) -> sVcCexv_D_ExvPosnReq2FEnaState/1
  TmOut/60(sVcEexv_D_ExvCal2FEnaState) -> sVcEexv_D_ExvCal2FEnaState/1

== system ScriptDemo/Create/creatIFOut/Before ==
